simulink model "diagramaDeBloques"  (R2025b)
settings: Solver=VariableStepAuto  StartTime=0.0  StopTime=0  RelTol=1e-3
InitFcn:
  | %% =========================================================
  | %  BAND-PASS
  | %
  | %                    -Rf*Cin*s
  | % Hbp(s) = ----------------------------------------
  | %          Rin*Rf*Cin*Cf*s^2 + (Rin*Cin+Rf*Cf)*s + 1
  | %% =========================================================
  | 
  | Rin_bp = 43e3;                  % Ohm
  | Rf_bp  = 43e3;                  % Ohm
  | Cin_bp = 680e-6;                % F
  | Cf_bp  = (150 + 27)*1e-12;      % F = 177 pF
  | 
  | % Numerador: -Rf*Cin*s + 0
  | num_Hbp = [-Rf_bp*Cin_bp, 0];
  | 
  | % Denominador: a2*s^2 + a1*s + a0
  | den_Hbp = [Rin_bp*Rf_bp*Cin_bp*Cf_bp, ...
  |            Rin_bp*Cin_bp + Rf_bp*Cf_bp, ...
  |            1];
  | 
  | 
  | 
  | 
  | %% =========================================================
  | %  LOW-PASS MULTIPLE FEEDBACK
  | %
  | %                         -(R2/R1)
  | % Hlp(s) = -------------------------------------------------
  | %          R2*R3*C1*C2*s^2 +
  | %          C2*(R2+R3+R2*R3/R1)*s + 1
  | %% =========================================================
  | 
  | R1_lp = 30e3;       % Ohm
  | R2_lp = 150e3;      % Ohm
  | R3_lp = 12e3;       % Ohm
  | C1_lp = 47e-9;      % F
  | C2_lp = 3.3e-9;     % F
  | 
  | % Numerador constante
  | num_Hlp = -(R2_lp/R1_lp);
  | 
  | % Denominador: a2*s^2 + a1*s + a0
  | den_Hlp = [R2_lp*R3_lp*C1_lp*C2_lp, ...
  |            C2_lp*(R2_lp + R3_lp + R2_lp*R3_lp/R1_lp), ...
  |            1];
  | 
  | 
  | 
  | 
  | %% Mostrar resultados
libraries: slctrl_linear x1
settings Model: Creator=elias  LastModifiedBy=elias

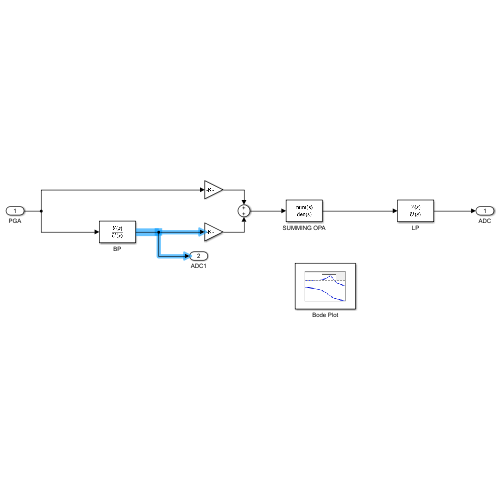
[thumbnail: Simulink's stored preview of the top-level diagram]
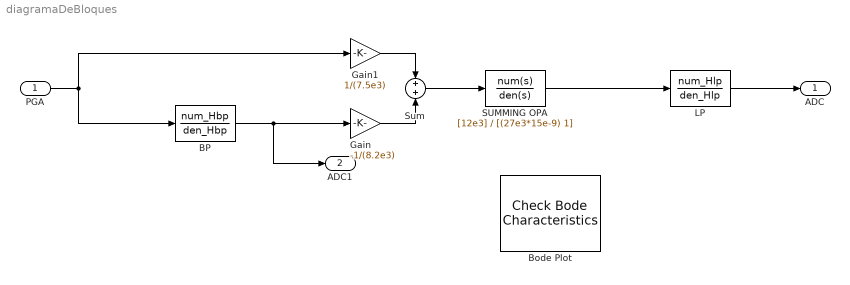
== system diagramaDeBloques ==
  PGA : Inport
  BP : TransferFcn  Numerator=num_Hbp  Denominator=den_Hbp
  Bode Plot : slctrl_linear/Check Bode  Characteristics  InstantiateOnLoad=on  SaveOperatingPoints=off  LinearizationIOs={'/PGA', 1, 'in', 'off', '';'/BP', 1, 'out', 'off', ''}  LinearizeAt=SnapshotTimes  SnapshotTimes=[0]  TriggerType=rising  SampleTime=auto  RateConversionMethod=zoh  PreWarpFreq=10  UseExactDelayModel=off  UseFullBlockNameLabels=off  UseBusSignalLabels=off  enabled=on  stopWhenAssertionFail=off  export=off  ViewDlgPos=[1 49 1920 960]  OpenViewOnLoad=on  LaunchViewOnOpen=off  FrequencyUnits=rad/s  MagnitudeUnits=dB  PhaseUnits=deg  TimeUnits=seconds  EnableUpperBound=off  UpperBoundFrequencies=[]  UpperBoundMagnitudes=[]  EnableLowerBound=off  LowerBoundFrequencies=[]  LowerBoundMagnitudes=[]
      settings: LibrarySourceBlock=slctrlblks/Linear Analysis Plots/Bode Plot  SaveToWorkspace=off  SaveName=sys
  Gain : Gain  Gain=-1/(8.2e3)
  Gain1 : Gain  Gain=1/(7.5e3)
  LP : TransferFcn  Numerator=num_Hlp  Denominator=den_Hlp
  SUMMING OPA : TransferFcn  Numerator=[12e3]  Denominator=[(27e3*15e-9) 1]
  Sum : Sum
  ADC : Outport
  ADC1 : Outport  Port=2
  wires:
  PGA/1 -> BP/1, Gain1/1
  BP/1 -> ADC1/1, Gain/1
  Gain1/1 -> Sum/1
  Gain/1 -> Sum/2
  Sum/1 -> SUMMING OPA/1
  SUMMING OPA/1 -> LP/1
  LP/1 -> ADC/1
